simulink model "simply54_1"  (R2021a)
settings: Solver=VariableStepAuto  StartTime=0.0  StopTime=10.0  RelTol=1e-3
libraries: simulink x6
settings Model: SimulationMode=accelerator  Creator=LENOVO  LastModifiedBy=CMelt

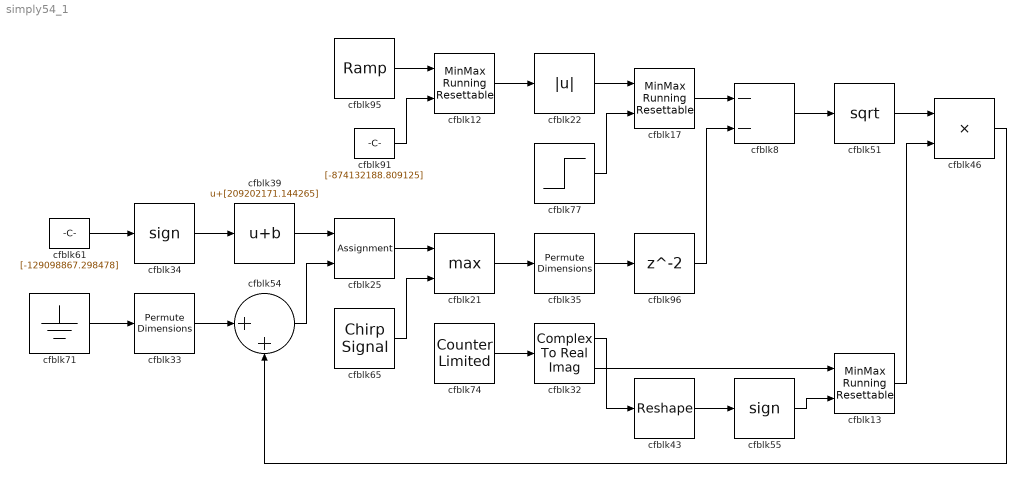
== system simply54_1 ==
  cfblk12 : simulink/Math Operations/MinMax Running Resettable  Function=min  vinit=0.0
  cfblk13 : simulink/Math Operations/MinMax Running Resettable  Function=min  vinit=0.0
  cfblk17 : simulink/Math Operations/MinMax Running Resettable  Function=min  vinit=0.0
  cfblk21 : MinMax  Function=max  Inputs=2
  cfblk22 : Abs
  cfblk25 : Assignment  DiagnosticForDimensions=Warning  IndexOptions=Index vector (dialog)  Indices=1  OutputSizes=1
  cfblk32 : ComplexToRealImag
  cfblk33 : PermuteDimensions
  cfblk34 : Signum
  cfblk35 : PermuteDimensions
  cfblk39 : Bias  Bias=[209202171.144265]
  cfblk43 : Reshape
  cfblk46 : Product
  cfblk51 : Sqrt  SaturateOnIntegerOverflow=on
  cfblk54 : Sum  Inputs=|++
  cfblk55 : Signum
  cfblk61 : Constant  Value=[-129098867.298478]  SampleTime=1
  cfblk65 : simulink/Sources/Chirp Signal  f1=[-916985926.712173]  T=[-126511661.542243]  f2=[360713620.554140]
  cfblk71 : Ground
  cfblk74 : simulink/Sources/Counter Limited  uplimit=[667.000000]  tsamp=-1
  cfblk77 : Step  Time=[36.000000]  Before=[989057779.543785]  After=[-46709576.045913]  SampleTime=0
  cfblk8 : Sum  Inputs=--
  cfblk91 : Constant  Value=[-874132188.809125]  SampleTime=1
  cfblk95 : simulink/Sources/Ramp  slope=[9920.536367]  start=[37.074568]  InitialOutput=[-885041.909920]
  cfblk96 : Delay  SampleTime=1
  wires:
  cfblk13/1 -> cfblk46/2
  cfblk12/1 -> cfblk22/1
  cfblk46/1 -> cfblk54/2
  cfblk32/1 -> cfblk43/1
  cfblk51/1 -> cfblk46/1
  cfblk33/1 -> cfblk54/1
  cfblk61/1 -> cfblk34/1
  cfblk17/1 -> cfblk8/1
  cfblk55/1 -> cfblk13/2
  cfblk21/1 -> cfblk35/1
  cfblk54/1 -> cfblk25/2
  cfblk43/1 -> cfblk55/1
  cfblk22/1 -> cfblk17/1
  cfblk77/1 -> cfblk17/2
  cfblk34/1 -> cfblk39/1
  cfblk65/1 -> cfblk21/2
  cfblk74/1 -> cfblk32/1
  cfblk95/1 -> cfblk12/1
  cfblk32/2 -> cfblk13/1
  cfblk25/1 -> cfblk21/1
  cfblk39/1 -> cfblk25/1
  cfblk35/1 -> cfblk96/1
  cfblk71/1 -> cfblk33/1
  cfblk96/1 -> cfblk8/2
  cfblk91/1 -> cfblk12/2
  cfblk8/1 -> cfblk51/1
